simulink model "zad6_test"  (R2022b)
settings: Solver=VariableStepAuto  StartTime=0.0  StopTime=10.0  RelTol=1e-3
undefined symbols (not defined in the file): a21, a23, a31, a33, b31, g, Kx, u0, x1, x2, x3, xd
settings Model: Creator=MPatr  LastModifiedBy=MPatr

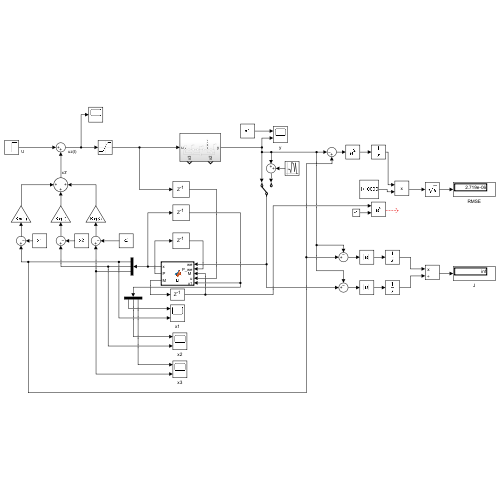
[thumbnail: Simulink's stored preview of the top-level diagram]
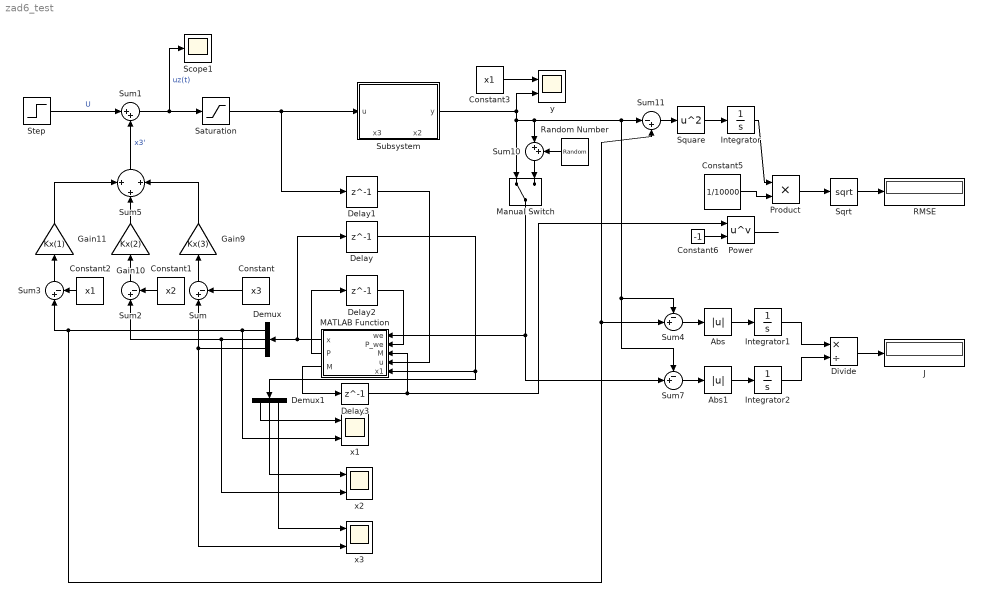
== system zad6_test ==
  Abs : Abs  SaturateOnIntegerOverflow=off
  Abs1 : Abs  SaturateOnIntegerOverflow=off
  Constant : Constant  Value=x3
  Constant1 : Constant  Value=x2
  Constant2 : Constant  Value=x1
  Constant3 : Constant  Value=x1
  Constant5 : Constant  Value=1/10000
  Constant6 : Constant  Value=-1
  Delay : Delay  DelayLength=1  InitialCondition=[xd; 0; 0]
  Delay1 : Delay  DelayLength=1  InitialCondition=0
  Delay2 : Delay  DelayLength=1  InitialCondition=[0 0 0; 0 0 0; 0 0 0]
  Delay3 : Delay  DelayLength=1  InitialCondition=0
  Demux : Demux  Outputs=3
  Demux1 : Demux  Outputs=3
  Divide : Product  Inputs=*/
  Gain10 : Gain  Gain=Kx(2)
  Gain11 : Gain  Gain=Kx(1)
  Gain9 : Gain  Gain=Kx(3)
  Integrator : Integrator
  Integrator1 : Integrator
  Integrator2 : Integrator
  J : Display
  MATLAB Function : MATLAB Function  TreatAsAtomicUnit=on
  Manual Switch : ManualSwitch
  Power : Math  Operator=pow
  Product : Product
  RMSE : Display
  Random Number : RandomNumber  Variance=.0000001
  Saturation : Saturate  UpperLimit=1  LowerLimit=0
  Scope1 : Scope
  Sqrt : Sqrt
  Square : Math  Operator=square
  Step : Step  Time=0  After=u0  SampleTime=0
  Subsystem : Subsystem
      settings: PortSchema="{\"entries\":[{\"content\":{\"sides\":[{\"content\":{\"connectorIds\":[\"In1\"]},\"type\":\"ConnectorPlacement.EquallySpacedRectSide\",\"uuid\":\"a9618e66-a868-4602-adbc-d46c199391e9\"},{\"content\":{\"connectorIds\":[\"Out1\"],\"side\":\"RIGHT\"},\"type\":\"ConnectorPlacement.EquallySpacedRectSide\",\"uuid\":\"c3196c58-25c5-4c17-9484-b8d421343e51\"},{\"content\":{\"connectorIds\":[],\"side\":\"TOP\"},\"type\":\"ConnectorPlacement.EquallySpacedRectSide\",\"uuid\":\"906d255b-3a1d-4e09-a9da-ed665958d266\"},{\"content\":{\"connectorIds\":[\"Out2\",\"Out3\"],\"side\":\"BOTTOM\"},\"type\":\"ConnectorPlacement.EquallySpacedRectSide\",\"uuid\":\"d9e5422d-f936-4847-a7ac-e53a1bad6272\"}]},\"type\":\"ConnectorPlacement.EquallySpacedConnector\",\"uuid\":\"1b3fe789-ebdd-4120-9cfb-1ec5ed381a45\"}],\"packageUris\":[\"http://schema.mathworks.com/mf0/Connector/R2020b\"],\"version\":\"1.0\"}"
  Sum : Sum  Inputs=|+-
  Sum1 : Sum  Inputs=|++
  Sum10 : Sum  Inputs=|++
  Sum11 : Sum  Inputs=|-+
  Sum2 : Sum  Inputs=|+-
  Sum3 : Sum  Inputs=|+-
  Sum4 : Sum  Inputs=-+|
  Sum5 : Sum  Inputs=+|+|+
  Sum7 : Sum  Inputs=-+|
  x1 : Scope  NumInputPorts=2
  x2 : Scope  NumInputPorts=2
  x3 : Scope  NumInputPorts=2
  y : Scope  NumInputPorts=2
  wires:
  Integrator1/1 -> Divide/1
  Demux/1 -> x1/2, Sum4/2, Sum11/2, Sum3/1
  Divide/1 -> J/1
  Constant6/1 -> Power/2
  Power/1 -> ?
  Constant5/1 -> Product/2
  Sum7/1 -> Abs1/1
  Sum/1 -> Gain9/1
  Sum11/1 -> Square/1
  Product/1 -> Sqrt/1
  Sum4/1 -> Abs/1
  MATLAB Function/3(M) -> Delay3/1
  Constant1/1 -> Sum2/2
  MATLAB Function/2(P) -> Delay2/1
  Demux/3 -> x3/2, Sum/1
  Demux1/1 -> x1/1
  Square/1 -> Integrator/1
  Demux1/2 -> x2/1
  Constant/1 -> Sum/2
  Constant2/1 -> Sum3/2
  Demux1/3 -> x3/1
  Delay1/1 -> MATLAB Function/4(u)
  Constant3/1 -> y/1
  Sum3/1 -> Gain11/1
  Delay3/1 -> MATLAB Function/3("M "), Power/1
  Integrator2/1 -> Divide/2
  Sum5/1 -> Sum1/2  "x3'"
  Abs1/1 -> Integrator2/1
  Integrator/1 -> Product/1
  Sum2/1 -> Gain10/1
  MATLAB Function/1(x) -> Demux/1, Delay/1
  Manual Switch/1 -> MATLAB Function/1(we), Sum7/2
  Abs/1 -> Integrator1/1
  Delay2/1 -> MATLAB Function/2(P_we)
  Gain11/1 -> Sum5/1
  Saturation/1 -> Delay1/1, Subsystem/1(u)
  Subsystem/1(y) -> Sum7/1, Sum4/1, Sum11/1, Sum10/1, Manual Switch/1, y/2
  Random Number/1 -> Sum10/2
  Sum10/1 -> Manual Switch/2
  Gain9/1 -> Sum5/3
  Sum1/1 -> Saturation/1, Scope1/1  "uz(t)"
  Delay/1 -> MATLAB Function/5(x1), Demux1/1
  Sqrt/1 -> RMSE/1
  Demux/2 -> Sum2/1, x2/2
  Step/1 -> Sum1/1  "U"
  Gain10/1 -> Sum5/2

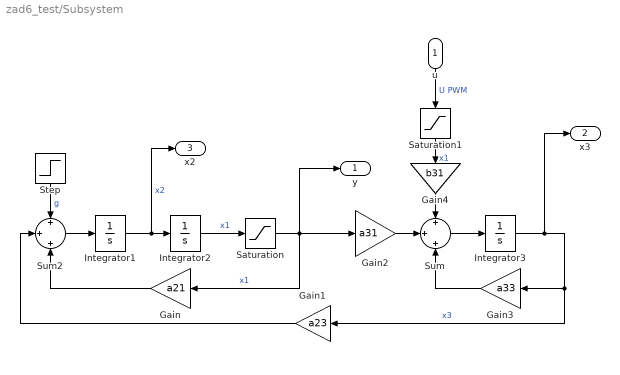
== system zad6_test/Subsystem ==
  u : Inport
  Gain : Gain  Gain=a21
  Gain1 : Gain  Gain=a23
  Gain2 : Gain  Gain=a31
  Gain3 : Gain  Gain=a33
  Gain4 : Gain  Gain=b31
  Integrator1 : Integrator
  Integrator2 : Integrator  InitialCondition=xd
  Integrator3 : Integrator
  Saturation : Saturate  UpperLimit=xd  LowerLimit=0
  Saturation1 : Saturate  UpperLimit=1  LowerLimit=0
  Step : Step  Time=0  After=g  SampleTime=0
  Sum : Sum  Inputs=+|+|+
  Sum2 : Sum  Inputs=+|+|+
  y : Outport
  x3 : Outport  Port=2
  x2 : Outport  Port=3
  wires:
  Step/1 -> Sum2/1  "g"
  Integrator1/1 -> x2/1, Integrator2/1  "x2"
  Gain1/1 -> Sum2/2
  u/1 -> Saturation1/1  "U PWM"
  Saturation/1 -> Gain/1, Gain2/1, y/1  "x1"
  Integrator3/1 -> x3/1, Gain1/1, Gain3/1  "x3"
  Gain/1 -> Sum2/3
  Gain2/1 -> Sum/2
  Gain3/1 -> Sum/3
  Sum2/1 -> Integrator1/1
  Sum/1 -> Integrator3/1
  Integrator2/1 -> Saturation/1  "x1"
  Gain4/1 -> Sum/1
  Saturation1/1 -> Gain4/1  "x1"

== matlab function zad6_test/MATLAB Function ==
  data: we input; x output; P output; P_we input; M input; M output; u input; x1 input
function [x, P, M]  = kf(we, P_we, M, u, x1)
%% Odczyt wejsc
y = we;  % aktualny pomiar

%% Parametry
m = .00575;
g = 9.81;
FemP1 = .017521;
FemP2 = .0058231;
f1 = .00014142;
f2 = .0045626;
ki = 2.5165;
ci = .0243 * sign(4-2);
d = .0792;
bd = .06;
xd = d-bd;
x10 = .008;
x20 = 0;
x30 = .75;
u10 = 1/ki*(x30-ci);

a21 = 1/(2*m)*x30^2*FemP1/FemP2^2*exp(-x10/FemP2); 
a23 = -1/(m)*x30*FemP1/FemP2*exp(-x10/FemP2); 
a31 = 1/f1*exp(x10/f2)*(ki*u10+ci-x30); 
a33 = -f2/f1*exp(x10/f2);
b31 = ki*f2/f1*exp(x10/f2);

% Do sprawdzenia zakłóceń wewnętrzynych
% A = [0 1 0; a21 0 a23; a31*1.01 0 a33*1.02];
A = [0 1 0; a21 0 a23; a31 0 a33];
B = [0 0; 0 g; b31 0];
C = [1 0 0];
D = 0;

%% Dyskretyzacja modelu metodą Eulera w przód(na podstawie instrukcji lab5)
Tp = 0.0001;
Ad = (eye(3)+A*Tp);
Bd = B*Tp;
Cd = C;
Dd = D;

%% Nastawy filtru
var_n = 0.001; % wariancja szumu pomiarowego
var_v = 0.1; % wariancje szumow wewnetrznych

Q = diag([var_v, var_v, var_v]);    % macierz kowariancji szumow wewnetrznych
R = diag(var_n);  	% macierz kowariancji szumow pomiarowych

%% Algorytm filtru Kalmana
% Etap predykcji
x_d = Ad*x1 + Bd*[u; 1];
P_d = Ad*P_we*Ad' + Q;

% Etap filtracji
K = P_d*Cd' * ((Cd*P_d*Cd' + R)^-1);
x_hat = x_d + K*(y - Cd*x_d);

% Przekazanie danych
x = x_hat;
P = (eye(3)-K*Cd)*P_d;
M = M + 1;
end
